simulink model "isothermalCSTR_LinearSS"  (R2017a)
settings: Solver=VariableStepAuto  StartTime=0.0  StopTime=500.0  RelTol=1e-3
values from neighbouring files (symbols this model uses):
  A = A_e(U_ss(idx,:), X_ss(idx,:))    [iso_cstr_main.m]
  B = B_e(U_ss(idx,:), X_ss(idx,:))    [iso_cstr_main.m]
  C = [0 0; 0 1]    [iso_cstr_main.m]    (also in iso_model.m = [1 0; 0 1])
  cA_e = X_ss(idx,1)    [iso_cstr_main.m]
  cB_e = X_ss(idx,2)    [iso_cstr_main.m]
  U_ss = U_ss(idx,1)    [iso_cstr_main.m]    (also in iso_model.m = U_ss(I)')
  y0 = [cA_e cB_e cC_e cD_e]    [iso_cstr_main.m]
settings Model: Creator=minhotmog  LastModifiedBy=minhotmog

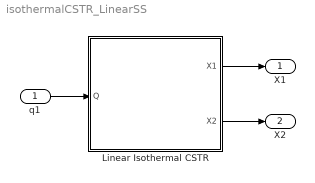
== system isothermalCSTR_LinearSS ==
  q1 : Inport
  Linear Isothermal CSTR : Subsystem
  X1 : Outport
  X2 : Outport  Port=2
  wires:
  Linear Isothermal CSTR/1(X1) -> X1/1
  Linear Isothermal CSTR/2(X2) -> X2/1
  q1/1 -> Linear Isothermal CSTR/1(Q)

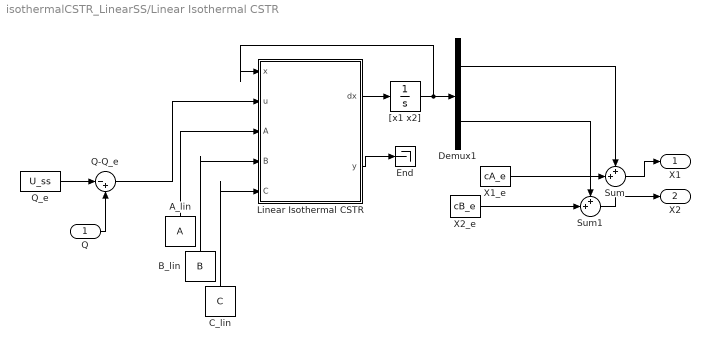
== system isothermalCSTR_LinearSS/Linear Isothermal CSTR ==
  Q : Inport
  A_lin : Constant  Value=A
  B_lin : Constant  Value=B
  C_lin : Constant  Value=C
  Demux1 : Demux  Outputs=2
  End : Terminator
  Linear Isothermal CSTR : MATLAB Function  TreatAsAtomicUnit=on
  Q-Q_e : Sum  Inputs=|-+
  Q_e : Constant  Value=U_ss
  Sum : Sum  Inputs=++|
  Sum1 : Sum  Inputs=++|
  X1_e : Constant  Value=cA_e
  X2_e : Constant  Value=cB_e
  "[x1 x2]" : Integrator  InitialCondition=[y0(1)-cA_e y0(2)-cB_e]  UpperSaturationLimit=[0.6 0.6 0.6]  LowerSaturationLimit=[0 0 0]
  X1 : Outport
  X2 : Outport  Port=2
  wires:
  Q-Q_e/1 -> Linear Isothermal CSTR/2(u)
  "[x1 x2]"/1 -> Linear Isothermal CSTR/1(x), Demux1/1
  Linear Isothermal CSTR/1(dx) -> "[x1 x2]"/1
  Q/1 -> Q-Q_e/2
  Q_e/1 -> Q-Q_e/1
  X1_e/1 -> Sum/2
  X2_e/1 -> Sum1/2
  A_lin/1 -> Linear Isothermal CSTR/3(A)
  Linear Isothermal CSTR/2(y) -> End/1
  B_lin/1 -> Linear Isothermal CSTR/4(B)
  C_lin/1 -> Linear Isothermal CSTR/5(C)
  Sum1/1 -> X2/1
  Sum/1 -> X1/1
  Demux1/2 -> Sum1/1
  Demux1/1 -> Sum/1

== matlab function isothermalCSTR_LinearSS/Linear Isothermal CSTR/Linear Isothermal CSTR ==
  data: x input; dx output; u input; y output; A input; B input; C input
function [dx, y] = Linear_SS(x, u, A, B, C)
    dx = zeros (2 ,1) ;
    y = zeros (2 ,1) ;
    
    dx = A * x + B * u;
    y  = C * x;
